simulink model "parte4_eje4_Tvapor"  (R2017b)
settings: Solver=VariableStepAuto  StartTime=0.0  StopTime=41  RelTol=1e-3
libraries: simulink x1
settings Model: Creator=Admon  LastModifiedBy=Admon

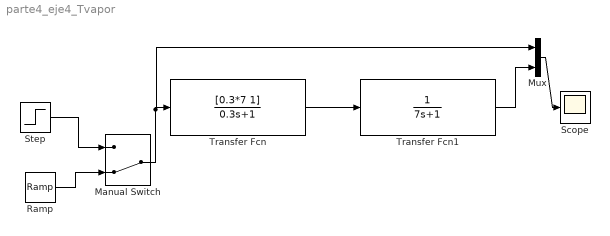
== system parte4_eje4_Tvapor ==
  Manual Switch : ManualSwitch  CurrentSetting=0
  Mux : Mux  Inputs=2
  Ramp : simulink/Sources/Ramp  slope=1  start=0  X0=0
  Scope : Scope
  Step : Step  SampleTime=0
  Transfer Fcn : TransferFcn  Numerator=[0.3*7 1]  Denominator=[0.3 1]
  Transfer Fcn1 : TransferFcn  Denominator=[7 1]
  wires:
  Transfer Fcn/1 -> Transfer Fcn1/1
  Step/1 -> Manual Switch/1
  Manual Switch/1 -> Mux/1, Transfer Fcn/1
  Ramp/1 -> Manual Switch/2
  Mux/1 -> Scope/1
  Transfer Fcn1/1 -> Mux/2
